simulink model "FaultedPMSM"  (R2023a)
settings: Solver=VariableStepAuto  StartTime=0.0  StopTime=1  MaxStep=1e-4  RelTol=1e-3  AbsTol=1e-3
PreLoadFcn:
  | FaultedPMSMParameters;
undefined symbols (not defined in the file or in its folder): J, RL, Rs, Rsl, Rw, Ry
libraries: fl_lib x45, ee_lib x19, nesl_utility x2
CloseFcn:
  | try close(h1_FaultedPMSM),end
  | clear h1_FaultedPMSM
  | 
  | clear B0    Ld    Npp   Nws   RL    Rsl   Ry
  | clear  g     gT    l     mu0   r     wS
  | clear J   Lq    Ns    PHI   Rs    Rw    csaT
  | clear gS    gY    lm    mur   rY    wY
  | clear gWinding L0 InitialRotorAnglePMSM
  | 
  | clear simlog_FaultedPMSM tout
Description:
  | PMSM with Thermal Model
settings Model: Creator=The MathWorks, Inc.  LastModifiedBy=Derrick Baalaboore
settings SolverCC: AutoScaleAbsTol=off  AlgebraicLoopSolver=TrustRegion
settings DataIOCC: MaxDataPoints=210000  SaveFormat=Array  ReturnWorkspaceOutputs=off  SignalLoggingName=logsout_PMSMWithThermal
settings OptimizationCC: BlockReduction=off  BooleanDataType=off  ReuseModelBlockBuffer=off  LifeSpan=inf
settings DebuggingCC: SaveWithParameterizedLinksMsg=none  UnderspecifiedInitializationDetection=Classic  MergeDetectMultiDrivingBlocksExec=none  SignalResolutionControl=TryResolveAllWithWarning  UnconnectedInputMsg=warning  UnconnectedOutputMsg=warning  UnconnectedLineMsg=warning  AllowSymbolicDim=off  SFUnexpectedBacktrackingDiag=warning  SFNoUnconditionalDefaultTransitionDiag=warning  SFExecutionAtInitializationDiag=none  ArithmeticOperatorsInVariantConditions=warning
settings HardwareCC: ProdBitPerPointer=32  ProdBitPerSizeT=32  ProdBitPerPtrDiffT=32  ProdLargestAtomicFloat=None  ProdIntDivRoundTo=Undefined  ProdEndianess=Unspecified  ProdWordSize=32  ProdHWDeviceType=32-bit Generic  TargetUnknown=on
settings ModelReferenceCC: EnableRefExpFcnMdlSchedulingChecks=on  PropagateSignalLabelsOutOfModel=off
settings SFSimCC: SimUseLocalCustomCode=off  CustomCodeUndefinedFunction=UseInterfaceOnly
settings RTWCC: RTWUseLocalCustomCode=off  DLArmComputeVersion=19.05
settings CodeAppCC: StateflowObjectComments=on
settings GRTTargetCC: TargetLangStandard=C89/C90 (ANSI)
settings ConfigComp: CovMetricSettings=dw  CovSaveCumulativeToWorkspaceVar=on  CovSaveSingleToWorkspaceVar=on  CovExternalEMLEnable=off  CovSFcnEnable=off
settings SimscapeCC: SimscapeLogType=all  SimscapeLogName=simlog_FaultedPMSM  SimscapeLogDecimation=10  SimscapeLogDataHistory=50000

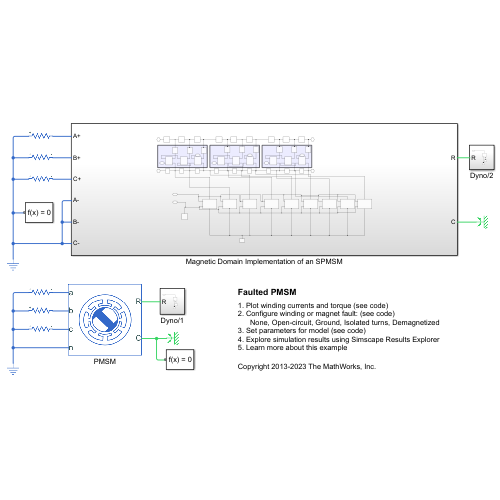
[thumbnail: Simulink's stored preview of the top-level diagram]
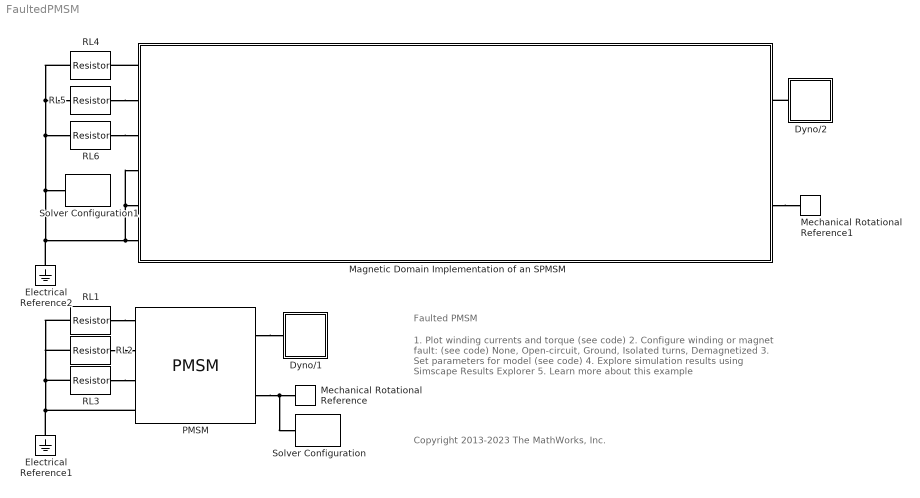
== system FaultedPMSM ==
  note: Faulted PMSM
  note: 1. Plot winding currents and torque (see code)
      | 2. Configure winding or magnet fault: (see code)
      |       None, Open-circuit, Ground, Isolated turns, Demagnetized
      | 3. Set parameters for model (see code)
      | 4. Explore simulation results using Simscape Results Explorer
      | 5. Learn more about this example
  note: Copyright 2013-2023 The MathWorks, Inc.
  Dyno/1 : Subsystem
  Dyno/2 : Subsystem
  Electrical Reference1 : fl_lib/Electrical/Electrical Elements/Electrical Reference
  Electrical Reference2 : fl_lib/Electrical/Electrical Elements/Electrical Reference
  Magnetic Domain Implementation of an SPMSM : Subsystem
  Mechanical Rotational Reference : fl_lib/Mechanical/Rotational Elements/Mechanical Rotational Reference
  Mechanical Rotational Reference1 : fl_lib/Mechanical/Rotational Elements/Mechanical Rotational Reference
  PMSM : ee_lib/Electromechanical/Permanent Magnet/PMSM  port_option=ee.enum.threePhasePort.expanded  winding_type=ee.enum.statorconnection.wye  machine_param=ee.enum.pmsm.parameterization.constant  nPolePairs=Npp  pmflux_param=ee.enum.pmflux.fluxlinkage  pm_flux_linkage=PHI Wb  torque_constant=0.18 N*m/A  back_emf_constant=0.18 V/(rad/s)  stator_param=ee.enum.statorparam.LdLqL0  Ld=Ld H  Lq=Lq H  idVec=[-200, 0, 200] A  iqVec=[-200, 0, 200] A  LdMatrix=0.0002 * ones(3, 3) H  LqMatrix=0.0002 * ones(3, 3) H  PmMatrix=0.1 * ones(3, 3) Wb  ktMatrix=0.18 * ones(3, 3) N*m/A  keMatrix=0.18 * ones(3, 3) V/(rad/s)  L0=L0 H  Ls=0.0002 H  Lm=-0.00002 H  Ms=0.00002 H  Rs=Rw Ohm  zero_sequence=ee.enum.park.zerosequence.include  axes_param=ee.enum.rotorangle.daxis  loss_param=ee.enum.ironloss.none  losses_oc=[0, 0, 0] W  losses_sc=[0, 0, 0] W  f_losses=60 Hz  Isc_losses=95 A  J=J kg*m^2  lam=0 N*m/(rad/s)  i_d_specify=off  i_d_priority=High  i_d=0 A  i_d_nominal_specify=off  i_d_nominal_unit=A  i_d_nominal_value=1  i_q_specify=off  i_q_priority=High  i_q=0 A  i_q_nominal_specify=off  i_q_nominal_unit=A  i_q_nominal_value=1  torque_specify=off  torque_priority=None  torque=0 N*m  torque_nominal_specify=off  torque_nominal_unit=N*m  torque_nominal_value=1  angular_velocity_specify=on  angular_velocity_priority=None  angular_velocity=0 rpm  angular_velocity_nominal_specify=off  angular_velocity_nominal_unit=rpm  angular_velocity_nominal_value=1  angular_position_specify=on  angular_position_priority=High  angular_position=InitialRotorAnglePMSM deg  angular_position_nominal_specify=off  angular_position_nominal_unit=deg  angular_position_nominal_value=1  alpha=3.93e-3 1/K  alpha_flux=-0.001 1/K  Tmeas=298.15 K  stator_thermal_mass=100 J/K  rotor_thermal_mass=200 J/K  Rm_percent_rotor=90  Rd_percent_rotor=30  temperatureA_specify=off  temperatureA_priority=High  temperatureA=25 degC  temperatureA_nominal_specify=off  temperatureA_nominal_unit=degC  temperatureA_nominal_value=1  temperatureB_specify=off  temperatureB_priority=High  temperatureB=25 degC  temperatureB_nominal_specify=off  temperatureB_nominal_unit=degC  temperatureB_nominal_value=1  temperatureC_specify=off  temperatureC_priority=High  temperatureC=25 degC  temperatureC_nominal_specify=off  temperatureC_nominal_unit=degC  temperatureC_nominal_value=1  temperatureR_specify=off  temperatureR_priority=High  temperatureR=25 degC  temperatureR_nominal_specify=off  temperatureR_nominal_unit=degC  temperatureR_nominal_value=1
      settings: InternalSimscapePortConfiguration="{\"Bottom\":[],\"Left\":[{\"id\":\"a\",\"label\":\"a\",\"type\":\"foundation.electrical.electrical\"},{\"id\":\"b\",\"label\":\"b\",\"type\":\"foundation.electrical.electrical\"},{\"id\":\"c\",\"label\":\"c\",\"type\":\"foundation.electrical.electrical\"},{\"id\":\"n\",\"label\":\"n\",\"type\":\"foundation.electrical.electrical\"}],\"Right\":[{\"id\":\"R\",\"label\":\"R\",\"type\":\"foundation.mechanical.rotational.rotational\"},{\"id\":\"C\",\"label\":\"C\",\"type\":\"foundation.mechanical.rotational.rotational\"}],\"Top\":[]}"
  RL1 : fl_lib/Electrical/Electrical Elements/Resistor  R=RL Ohm  i_specify=on  i_priority=High  i=0 A  i_nominal_specify=off  i_nominal_unit=A  i_nominal_value=1  v_specify=off  v_priority=None  v=0 V  v_nominal_specify=off  v_nominal_unit=V  v_nominal_value=1
  RL2 : fl_lib/Electrical/Electrical Elements/Resistor  R=RL Ohm  i_specify=on  i_priority=High  i=0 A  i_nominal_specify=off  i_nominal_unit=A  i_nominal_value=1  v_specify=off  v_priority=None  v=0 V  v_nominal_specify=off  v_nominal_unit=V  v_nominal_value=1
  RL3 : fl_lib/Electrical/Electrical Elements/Resistor  R=RL Ohm  i_specify=on  i_priority=High  i=0 A  i_nominal_specify=off  i_nominal_unit=A  i_nominal_value=1  v_specify=off  v_priority=None  v=0 V  v_nominal_specify=off  v_nominal_unit=V  v_nominal_value=1
  RL4 : fl_lib/Electrical/Electrical Elements/Resistor  R=RL Ohm  i_specify=off  i_priority=High  i=0 A  i_nominal_specify=off  i_nominal_unit=A  i_nominal_value=1  v_specify=off  v_priority=None  v=0 V  v_nominal_specify=off  v_nominal_unit=V  v_nominal_value=1
  RL5 : fl_lib/Electrical/Electrical Elements/Resistor  R=RL Ohm  i_specify=off  i_priority=High  i=0 A  i_nominal_specify=off  i_nominal_unit=A  i_nominal_value=1  v_specify=off  v_priority=None  v=0 V  v_nominal_specify=off  v_nominal_unit=V  v_nominal_value=1
  RL6 : fl_lib/Electrical/Electrical Elements/Resistor  R=RL Ohm  i_specify=off  i_priority=High  i=0 A  i_nominal_specify=off  i_nominal_unit=A  i_nominal_value=1  v_specify=off  v_priority=None  v=0 V  v_nominal_specify=off  v_nominal_unit=V  v_nominal_value=1
  Solver Configuration : nesl_utility/Solver Configuration  PhysicalDomain=network_engine_domain  SubClassName=solver  LeftPortType=input  RightPortType=generic  Tones=[]  Harmonics=[]  SimulateNoise=off  Profile=off  UseLocalSampling=off  EnableSwitchedLinearOptims=on  FrequencyDomain=off  UseCCode=off  RelTol=0.001  AbsTol=1e-06  MinStep=1e-09  ToWorkspace=off  RevertToSquareIcSolve=off  NumHomotopyIterations=100  PhasorMode=off  PhasorModeNumHarmonics=1  ConsistencySolver=NEWTON_FTOL  IndexReductionMethod=DerivativeReplacement  DoDC=off  ResidualTolerance=1e-09  ConsistencyTolSource=GLOBAL  ConsistencyAbsTol=0.001  ConsistencyRelTol=0.001  ConsistencyTolFactor=0.001  UseLocalSolver=off  LocalSolverChoice=NE_BACKWARD_EULER_ADVANCER  ResolveIndetEquations=on  FunctionEvalNumThread=1  LocalSolverSampleTime=0.0001  DoFixedCost=off  MaxNonlinIter=3  MaxModeIter=2  ComputeImpulses=off  ImpulseIterations=1  LinearAlgebra=auto  LinearAlgebraNumThread=0  EquationFormulation=NE_TIME_EF  DelaysMemoryBudget=1024  AutomaticFiltering=on  FilteringTimeConstant=0.001  PartitionStorageMethod=AS_NEEDED  PartitionMemoryBudget=1024  PartitionMethod=ROBUST
  Solver Configuration1 : nesl_utility/Solver Configuration  PhysicalDomain=network_engine_domain  SubClassName=solver  LeftPortType=input  RightPortType=generic  Tones=[]  Harmonics=[]  SimulateNoise=off  Profile=off  UseLocalSampling=off  EnableSwitchedLinearOptims=on  FrequencyDomain=off  UseCCode=off  RelTol=0.001  AbsTol=1e-06  MinStep=1e-09  ToWorkspace=off  RevertToSquareIcSolve=off  NumHomotopyIterations=100  PhasorMode=off  PhasorModeNumHarmonics=1  ConsistencySolver=NEWTON_FTOL  IndexReductionMethod=DerivativeReplacement  DoDC=off  ResidualTolerance=1e-09  ConsistencyTolSource=GLOBAL  ConsistencyAbsTol=0.001  ConsistencyRelTol=0.001  ConsistencyTolFactor=0.001  UseLocalSolver=off  LocalSolverChoice=NE_BACKWARD_EULER_ADVANCER  ResolveIndetEquations=on  FunctionEvalNumThread=1  LocalSolverSampleTime=0.0001  DoFixedCost=off  MaxNonlinIter=3  MaxModeIter=2  ComputeImpulses=off  ImpulseIterations=1  LinearAlgebra=auto  LinearAlgebraNumThread=0  EquationFormulation=NE_TIME_EF  DelaysMemoryBudget=1024  AutomaticFiltering=on  FilteringTimeConstant=0.001  PartitionStorageMethod=AS_NEEDED  PartitionMemoryBudget=1024  PartitionMethod=ROBUST
  connections:
  Electrical Reference1/LConn1 -- PMSM/LConn4 -- RL1/LConn1 -- RL2/LConn1 -- RL3/LConn1
  PMSM/RConn1 -- Dyno/1/LConn1
  RL1/RConn1 -- PMSM/LConn1
  Magnetic Domain Implementation of an SPMSM/RConn2 -- Mechanical Rotational Reference1/LConn1
  RL3/RConn1 -- PMSM/LConn3
  Magnetic Domain Implementation of an SPMSM/LConn1 -- RL4/RConn1
  Dyno/2/LConn1 -- Magnetic Domain Implementation of an SPMSM/RConn1
  PMSM/RConn2 -- Solver Configuration/RConn1 -- Mechanical Rotational Reference/LConn1
  RL2/RConn1 -- PMSM/LConn2
  RL6/RConn1 -- Magnetic Domain Implementation of an SPMSM/LConn3
  RL5/RConn1 -- Magnetic Domain Implementation of an SPMSM/LConn2
  RL4/LConn1 -- Solver Configuration1/RConn1 -- Electrical Reference2/LConn1 -- Magnetic Domain Implementation of an SPMSM/LConn5 -- Magnetic Domain Implementation of an SPMSM/LConn4 -- Magnetic Domain Implementation of an SPMSM/LConn6 -- RL6/LConn1 -- RL5/LConn1

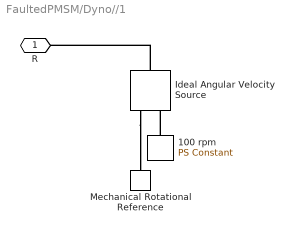
== system FaultedPMSM/Dyno//1 ==
  100 rpm : fl_lib/Physical Signals/Sources/PS Constant  constant=100 rpm
  Ideal Angular Velocity Source : fl_lib/Mechanical/Mechanical Sources/Ideal Angular Velocity Source
  Mechanical Rotational Reference : fl_lib/Mechanical/Rotational Elements/Mechanical Rotational Reference
  R : PMIOPort  Side=Left
  connections:
  Ideal Angular Velocity Source/RConn2 -- Mechanical Rotational Reference/LConn1
  Ideal Angular Velocity Source/LConn1 -- R/RConn1
  100 rpm/RConn1 -- Ideal Angular Velocity Source/RConn1

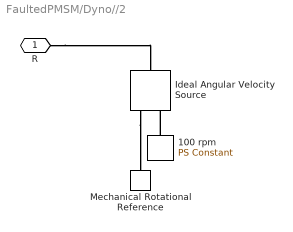
== system FaultedPMSM/Dyno//2 ==
  100 rpm : fl_lib/Physical Signals/Sources/PS Constant  constant=100 rpm
  Ideal Angular Velocity Source : fl_lib/Mechanical/Mechanical Sources/Ideal Angular Velocity Source
  Mechanical Rotational Reference : fl_lib/Mechanical/Rotational Elements/Mechanical Rotational Reference
  R : PMIOPort  Side=Left
  connections:
  100 rpm/RConn1 -- Ideal Angular Velocity Source/RConn1
  Ideal Angular Velocity Source/RConn2 -- Mechanical Rotational Reference/LConn1
  R/RConn1 -- Ideal Angular Velocity Source/LConn1

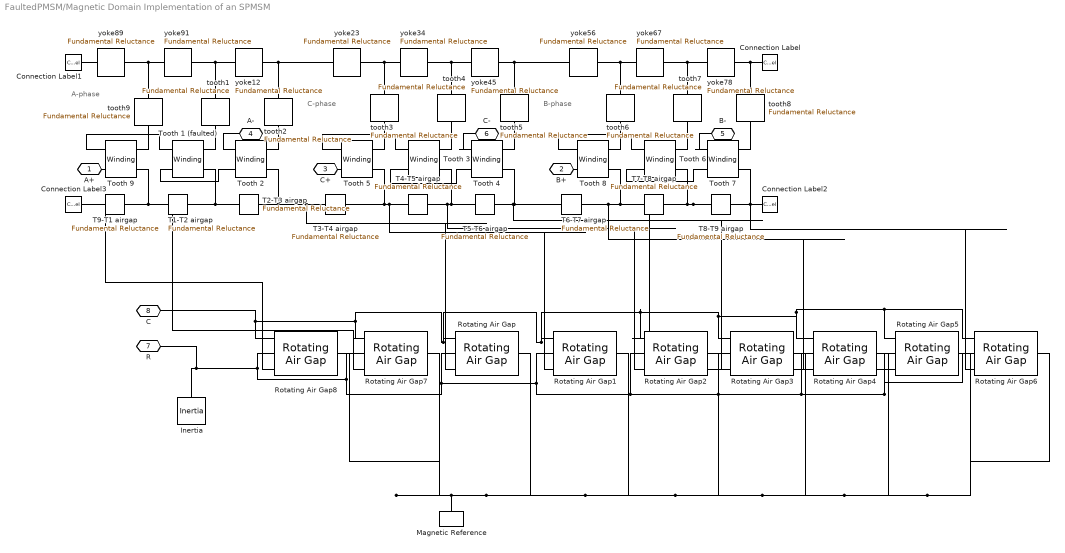
== system FaultedPMSM/Magnetic Domain Implementation of an SPMSM ==
  note: A-phase
  note: C-phase
  note: B-phase
  Connection Label : ConnectionLabel  Label=Y
  Connection Label1 : ConnectionLabel  Label=Y
  Connection Label2 : ConnectionLabel  Label=SL
  Connection Label3 : ConnectionLabel  Label=SL
  Inertia : fl_lib/Mechanical/Rotational Elements/Inertia  inertia=J kg*m^2  num_ports=foundation.enum.numPorts2.one  w_specify=on  w_priority=None  w=0 rad/s  w_nominal_specify=off  w_nominal_unit=rad/s  w_nominal_value=1  t_specify=off  t_priority=High  t=0 N*m  t_nominal_specify=off  t_nominal_unit=N*m  t_nominal_value=1
  Magnetic Reference : fl_lib/Magnetic/Magnetic Elements/Magnetic Reference
      settings: InternalSimscapePortConfiguration="{\"Bottom\":[],\"Left\":[{\"id\":\"M\",\"label\":\"\",\"type\":\"foundation.magnetic.magnetic\"}],\"Right\":[],\"Top\":[]}"
  Rotating Air Gap{,1..8} (9 alike) : ee_lib/Electromechanical/Rotating Air Gap  Nr=5  Ns=9  slot=1  B0=0.4 T  lm=5 mm  mur=1.05  g=1 mm  r=65 mm  l=50 mm  enable_faults=false  lambdaVec=ones(1, 10)  t_fault_transition=100 s  t_fault=1 s  mmf_specify=off  mmf_priority=None  mmf=0 A  mmf_nominal_specify=off  mmf_nominal_unit=A  mmf_nominal_value=1  phi_specify=off  phi_priority=None  phi=0 Wb  phi_nominal_specify=off  phi_nominal_unit=Wb  phi_nominal_value=1  t_specify=off  t_priority=None  t=0 N*m  t_nominal_specify=off  t_nominal_unit=N*m  t_nominal_value=1  w_specify=off  w_priority=None  w=0 rad/s  w_nominal_specify=off  w_nominal_unit=rad/s  w_nominal_value=1  rotorAngle_specify=off  rotorAngle_priority=High  rotorAngle=0 deg  rotorAngle_nominal_specify=off  rotorAngle_nominal_unit=deg  rotorAngle_nominal_value=1
      settings: InternalSimscapePortConfiguration="{\"Bottom\":[{\"id\":\"S\",\"label\":\"S\",\"type\":\"foundation.magnetic.magnetic\"}],\"Left\":[{\"id\":\"C\",\"label\":\"C\",\"type\":\"foundation.mechanical.rotational.rotational\"},{\"id\":\"R\",\"label\":\"R\",\"type\":\"foundation.mechanical.rotational.rotational\"}],\"Right\":[],\"Top\":[{\"id\":\"N\",\"label\":\"N\",\"type\":\"foundation.magnetic.magnetic\"}]}"
  T1-T2 airgap : fl_lib/Magnetic/Magnetic Elements/Fundamental Reluctance  R=Rsl 1/H  phi_specify=off  phi_priority=None  phi=0 Wb  phi_nominal_specify=off  phi_nominal_unit=Wb  phi_nominal_value=1  mmf_specify=off  mmf_priority=None  mmf=0 A  mmf_nominal_specify=off  mmf_nominal_unit=A  mmf_nominal_value=1
      settings: InternalSimscapePortConfiguration="{\"Bottom\":[],\"Left\":[{\"id\":\"N\",\"label\":\"N\",\"type\":\"foundation.magnetic.magnetic\"}],\"Right\":[{\"id\":\"S\",\"label\":\"S\",\"type\":\"foundation.magnetic.magnetic\"}],\"Top\":[]}"
  T2-T3 airgap : fl_lib/Magnetic/Magnetic Elements/Fundamental Reluctance  R=Rsl 1/H  phi_specify=off  phi_priority=None  phi=0 Wb  phi_nominal_specify=off  phi_nominal_unit=Wb  phi_nominal_value=1  mmf_specify=off  mmf_priority=None  mmf=0 A  mmf_nominal_specify=off  mmf_nominal_unit=A  mmf_nominal_value=1
      settings: InternalSimscapePortConfiguration="{\"Bottom\":[],\"Left\":[{\"id\":\"N\",\"label\":\"N\",\"type\":\"foundation.magnetic.magnetic\"}],\"Right\":[{\"id\":\"S\",\"label\":\"S\",\"type\":\"foundation.magnetic.magnetic\"}],\"Top\":[]}"
  T3-T4 airgap : fl_lib/Magnetic/Magnetic Elements/Fundamental Reluctance  R=Rsl 1/H  phi_specify=off  phi_priority=None  phi=0 Wb  phi_nominal_specify=off  phi_nominal_unit=Wb  phi_nominal_value=1  mmf_specify=off  mmf_priority=None  mmf=0 A  mmf_nominal_specify=off  mmf_nominal_unit=A  mmf_nominal_value=1
      settings: InternalSimscapePortConfiguration="{\"Bottom\":[],\"Left\":[{\"id\":\"N\",\"label\":\"N\",\"type\":\"foundation.magnetic.magnetic\"}],\"Right\":[{\"id\":\"S\",\"label\":\"S\",\"type\":\"foundation.magnetic.magnetic\"}],\"Top\":[]}"
  T4-T5 airgap : fl_lib/Magnetic/Magnetic Elements/Fundamental Reluctance  R=Rsl 1/H  phi_specify=off  phi_priority=None  phi=0 Wb  phi_nominal_specify=off  phi_nominal_unit=Wb  phi_nominal_value=1  mmf_specify=off  mmf_priority=None  mmf=0 A  mmf_nominal_specify=off  mmf_nominal_unit=A  mmf_nominal_value=1
      settings: InternalSimscapePortConfiguration="{\"Bottom\":[],\"Left\":[{\"id\":\"N\",\"label\":\"N\",\"type\":\"foundation.magnetic.magnetic\"}],\"Right\":[{\"id\":\"S\",\"label\":\"S\",\"type\":\"foundation.magnetic.magnetic\"}],\"Top\":[]}"
  T5-T6 airgap : fl_lib/Magnetic/Magnetic Elements/Fundamental Reluctance  R=Rsl 1/H  phi_specify=off  phi_priority=None  phi=0 Wb  phi_nominal_specify=off  phi_nominal_unit=Wb  phi_nominal_value=1  mmf_specify=off  mmf_priority=None  mmf=0 A  mmf_nominal_specify=off  mmf_nominal_unit=A  mmf_nominal_value=1
      settings: InternalSimscapePortConfiguration="{\"Bottom\":[],\"Left\":[{\"id\":\"N\",\"label\":\"N\",\"type\":\"foundation.magnetic.magnetic\"}],\"Right\":[{\"id\":\"S\",\"label\":\"S\",\"type\":\"foundation.magnetic.magnetic\"}],\"Top\":[]}"
  T6-T7 airgap : fl_lib/Magnetic/Magnetic Elements/Fundamental Reluctance  R=Rsl 1/H  phi_specify=off  phi_priority=None  phi=0 Wb  phi_nominal_specify=off  phi_nominal_unit=Wb  phi_nominal_value=1  mmf_specify=off  mmf_priority=None  mmf=0 A  mmf_nominal_specify=off  mmf_nominal_unit=A  mmf_nominal_value=1
      settings: InternalSimscapePortConfiguration="{\"Bottom\":[],\"Left\":[{\"id\":\"N\",\"label\":\"N\",\"type\":\"foundation.magnetic.magnetic\"}],\"Right\":[{\"id\":\"S\",\"label\":\"S\",\"type\":\"foundation.magnetic.magnetic\"}],\"Top\":[]}"
  T7-T8 airgap : fl_lib/Magnetic/Magnetic Elements/Fundamental Reluctance  R=Rsl 1/H  phi_specify=off  phi_priority=None  phi=0 Wb  phi_nominal_specify=off  phi_nominal_unit=Wb  phi_nominal_value=1  mmf_specify=off  mmf_priority=None  mmf=0 A  mmf_nominal_specify=off  mmf_nominal_unit=A  mmf_nominal_value=1
      settings: InternalSimscapePortConfiguration="{\"Bottom\":[],\"Left\":[{\"id\":\"N\",\"label\":\"N\",\"type\":\"foundation.magnetic.magnetic\"}],\"Right\":[{\"id\":\"S\",\"label\":\"S\",\"type\":\"foundation.magnetic.magnetic\"}],\"Top\":[]}"
  T8-T9 airgap : fl_lib/Magnetic/Magnetic Elements/Fundamental Reluctance  R=Rsl 1/H  phi_specify=off  phi_priority=None  phi=0 Wb  phi_nominal_specify=off  phi_nominal_unit=Wb  phi_nominal_value=1  mmf_specify=off  mmf_priority=None  mmf=0 A  mmf_nominal_specify=off  mmf_nominal_unit=A  mmf_nominal_value=1
      settings: InternalSimscapePortConfiguration="{\"Bottom\":[],\"Left\":[{\"id\":\"N\",\"label\":\"N\",\"type\":\"foundation.magnetic.magnetic\"}],\"Right\":[{\"id\":\"S\",\"label\":\"S\",\"type\":\"foundation.magnetic.magnetic\"}],\"Top\":[]}"
  T9-T1 airgap : fl_lib/Magnetic/Magnetic Elements/Fundamental Reluctance  R=Rsl 1/H  phi_specify=off  phi_priority=None  phi=0 Wb  phi_nominal_specify=off  phi_nominal_unit=Wb  phi_nominal_value=1  mmf_specify=off  mmf_priority=None  mmf=0 A  mmf_nominal_specify=off  mmf_nominal_unit=A  mmf_nominal_value=1
      settings: InternalSimscapePortConfiguration="{\"Bottom\":[],\"Left\":[{\"id\":\"N\",\"label\":\"N\",\"type\":\"foundation.magnetic.magnetic\"}],\"Right\":[{\"id\":\"S\",\"label\":\"S\",\"type\":\"foundation.magnetic.magnetic\"}],\"Top\":[]}"
  Tooth 1 (faulted) : ee_lib/Passive/Winding  Nw=Nws  Rw=Rw/3 Ohm  Rl=inf 1/H  Gw=gWinding 1/Ohm  thermalPort=simscape.enum.thermaleffects.omit  alpha=3.93e-3 1/K  Tmeas=25 degC  winding_thermal_mass=100 J/K  enable_faults=ee.enum.enable.no  fault_action=simscape.enum.assert.action.none  lambdaPercent=50  turnsShort=ee.enum.faults.faultTurnsShort.no  openCct=ee.enum.faults.faultTurnsOpenCkt.no  groundShort=ee.enum.faults.faultTurnsGroundShort.no  groundShortG=1000 1/Ohm  tau_fault=1e-3 s  fault_trigger=ee.enum.faults.faultTrigger.temporal  t_fault=0.5 s  max_permissible_voltage=100 V  n_fail_on_voltage=1  max_permissible_current=1 A  t_fail_on_current=1 s  T_specify=off  T_priority=None  T=25 degC  T_nominal_specify=off  T_nominal_unit=degC  T_nominal_value=1  i_specify=off  i_priority=None  i=0 A  i_nominal_specify=off  i_nominal_unit=A  i_nominal_value=1  v_specify=off  v_priority=High  v=0 V  v_nominal_specify=off  v_nominal_unit=V  v_nominal_value=1  phi_specify=off  phi_priority=None  phi=0 Wb  phi_nominal_specify=off  phi_nominal_unit=Wb  phi_nominal_value=1  faulted_specify=off  faulted_priority=None  faulted=0  iterm_p_specify=off  iterm_p_priority=None  iterm_p=0 A  iterm_p_nominal_specify=off  iterm_p_nominal_unit=A  iterm_p_nominal_value=1  iterm_n_specify=off  iterm_n_priority=None  iterm_n=0 A  iterm_n_nominal_specify=off  iterm_n_nominal_unit=A  iterm_n_nominal_value=1  power_dissipated_specify=off  power_dissipated_priority=None  power_dissipated=0 W  power_dissipated_nominal_specify=off  power_dissipated_nominal_unit=W  power_dissipated_nominal_value=1
      settings: InternalSimscapePortConfiguration="{\"Bottom\":[],\"Left\":[{\"id\":\"p\",\"label\":\"+\",\"type\":\"foundation.electrical.electrical\"},{\"id\":\"n\",\"label\":\"-\",\"type\":\"foundation.electrical.electrical\"}],\"Right\":[{\"id\":\"N\",\"label\":\"N\",\"type\":\"foundation.magnetic.magnetic\"},{\"id\":\"S\",\"label\":\"S\",\"type\":\"foundation.magnetic.magnetic\"}],\"Top\":[]}"
  Tooth {2..9} (8 alike) : ee_lib/Passive/Winding  Nw=Nws  Rw=Rw/3 Ohm  Rl=inf 1/H  Gw=gWinding 1/Ohm  thermalPort=simscape.enum.thermaleffects.omit  alpha=3.93e-3 1/K  Tmeas=25 degC  winding_thermal_mass=100 J/K  enable_faults=ee.enum.enable.no  fault_action=simscape.enum.assert.action.none  lambdaPercent=50  turnsShort=ee.enum.faults.faultTurnsShort.no  openCct=ee.enum.faults.faultTurnsOpenCkt.no  groundShort=ee.enum.faults.faultTurnsGroundShort.no  groundShortG=0 1/Ohm  tau_fault=1e-3 s  fault_trigger=ee.enum.faults.faultTrigger.temporal  t_fault=1 s  max_permissible_voltage=100 V  n_fail_on_voltage=1  max_permissible_current=1 A  t_fail_on_current=1 s  T_specify=off  T_priority=None  T=25 degC  T_nominal_specify=off  T_nominal_unit=degC  T_nominal_value=1  i_specify=off  i_priority=None  i=0 A  i_nominal_specify=off  i_nominal_unit=A  i_nominal_value=1  v_specify=off  v_priority=None  v=0 V  v_nominal_specify=off  v_nominal_unit=V  v_nominal_value=1  phi_specify=off  phi_priority=None  phi=0 Wb  phi_nominal_specify=off  phi_nominal_unit=Wb  phi_nominal_value=1  faulted_specify=off  faulted_priority=None  faulted=0  iterm_p_specify=off  iterm_p_priority=None  iterm_p=0 A  iterm_p_nominal_specify=off  iterm_p_nominal_unit=A  iterm_p_nominal_value=1  iterm_n_specify=off  iterm_n_priority=None  iterm_n=0 A  iterm_n_nominal_specify=off  iterm_n_nominal_unit=A  iterm_n_nominal_value=1  power_dissipated_specify=off  power_dissipated_priority=None  power_dissipated=0 W  power_dissipated_nominal_specify=off  power_dissipated_nominal_unit=W  power_dissipated_nominal_value=1
      settings: InternalSimscapePortConfiguration="{\"Bottom\":[],\"Left\":[{\"id\":\"p\",\"label\":\"+\",\"type\":\"foundation.electrical.electrical\"},{\"id\":\"n\",\"label\":\"-\",\"type\":\"foundation.electrical.electrical\"}],\"Right\":[{\"id\":\"N\",\"label\":\"N\",\"type\":\"foundation.magnetic.magnetic\"},{\"id\":\"S\",\"label\":\"S\",\"type\":\"foundation.magnetic.magnetic\"}],\"Top\":[]}"
  tooth{1..9} (9 alike) : fl_lib/Magnetic/Magnetic Elements/Fundamental Reluctance  R=Rs 1/H  phi_specify=off  phi_priority=None  phi=0 Wb  phi_nominal_specify=off  phi_nominal_unit=Wb  phi_nominal_value=1  mmf_specify=off  mmf_priority=None  mmf=0 A  mmf_nominal_specify=off  mmf_nominal_unit=A  mmf_nominal_value=1
      settings: InternalSimscapePortConfiguration="{\"Bottom\":[],\"Left\":[{\"id\":\"N\",\"label\":\"N\",\"type\":\"foundation.magnetic.magnetic\"}],\"Right\":[{\"id\":\"S\",\"label\":\"S\",\"type\":\"foundation.magnetic.magnetic\"}],\"Top\":[]}"
  yoke{12,23,34,45,56,67,78,89,91} (9 alike) : fl_lib/Magnetic/Magnetic Elements/Fundamental Reluctance  R=Ry 1/H  phi_specify=off  phi_priority=None  phi=0 Wb  phi_nominal_specify=off  phi_nominal_unit=Wb  phi_nominal_value=1  mmf_specify=off  mmf_priority=None  mmf=0 A  mmf_nominal_specify=off  mmf_nominal_unit=A  mmf_nominal_value=1
      settings: InternalSimscapePortConfiguration="{\"Bottom\":[],\"Left\":[{\"id\":\"N\",\"label\":\"N\",\"type\":\"foundation.magnetic.magnetic\"}],\"Right\":[{\"id\":\"S\",\"label\":\"S\",\"type\":\"foundation.magnetic.magnetic\"}],\"Top\":[]}"
  A+ : PMIOPort  Side=Left
  B+ : PMIOPort  Port=2  Side=Left
  C+ : PMIOPort  Port=3  Side=Left
  A- : PMIOPort  Port=4  Side=Left
  B- : PMIOPort  Port=5  Side=Left
  C- : PMIOPort  Port=6  Side=Left
  R : PMIOPort  Port=7  Side=Right
  C : PMIOPort  Port=8  Side=Right
  connections:
  yoke91/RConn1 -- yoke12/LConn1 -- tooth1/LConn1
  Tooth 1 (faulted)/RConn2 -- Rotating Air Gap7/LConn3 -- T2-T3 airgap/LConn1 -- T1-T2 airgap/RConn1
  Tooth 2/RConn1 -- tooth2/RConn1
  yoke91/LConn1 -- yoke89/RConn1 -- tooth9/LConn1
  yoke89/LConn1 -- Connection Label1/LConn1
  T9-T1 airgap/LConn1 -- Connection Label3/LConn1
  Tooth 9/LConn2 -- A+/RConn1
  Tooth 9/LConn1 -- Tooth 1 (faulted)/LConn1
  Tooth 1 (faulted)/LConn2 -- Tooth 2/LConn2
  Tooth 2/LConn1 -- A-/RConn1
  Tooth 9/RConn2 -- Rotating Air Gap8/LConn3 -- T9-T1 airgap/RConn1 -- T1-T2 airgap/LConn1
  yoke45/LConn1 -- yoke34/RConn1 -- tooth4/LConn1
  yoke34/LConn1 -- yoke23/RConn1 -- tooth3/LConn1
  yoke45/RConn1 -- yoke56/LConn1 -- tooth5/LConn1
  Tooth 5/LConn2 -- C+/RConn1
  Tooth 3/LConn2 -- Tooth 4/LConn2
  Tooth 5/LConn1 -- Tooth 3/LConn1
  Tooth 4/LConn1 -- C-/RConn1
  yoke78/LConn1 -- yoke67/RConn1 -- tooth7/LConn1
  Tooth 6/RConn2 -- T7-T8 airgap/RConn1 -- Rotating Air Gap5/LConn3 -- T8-T9 airgap/LConn1
  yoke67/LConn1 -- yoke56/RConn1 -- tooth6/LConn1
  tooth8/LConn1 -- yoke78/RConn1 -- Connection Label/LConn1
  Tooth 8/LConn2 -- B+/RConn1
  Tooth 8/LConn1 -- Tooth 6/LConn1
  Tooth 6/LConn2 -- Tooth 7/LConn2
  Tooth 7/LConn1 -- B-/RConn1
  Tooth 1 (faulted)/RConn1 -- tooth1/RConn1
  yoke23/LConn1 -- tooth2/LConn1 -- yoke12/RConn1
  Tooth 5/RConn1 -- tooth3/RConn1
  Tooth 3/RConn1 -- tooth4/RConn1
  Tooth 4/RConn1 -- tooth5/RConn1
  Tooth 8/RConn1 -- tooth6/RConn1
  Tooth 6/RConn1 -- tooth7/RConn1
  Tooth 9/RConn1 -- tooth9/RConn1
  Tooth 7/RConn1 -- tooth8/RConn1
  Magnetic Reference/LConn1 -- Rotating Air Gap6/RConn1 -- Rotating Air Gap5/RConn1 -- Rotating Air Gap4/RConn1 -- Rotating Air Gap3/RConn1 -- Rotating Air Gap2/RConn1 -- Rotating Air Gap1/RConn1 -- Rotating Air Gap/RConn1 -- Rotating Air Gap7/RConn1 -- Rotating Air Gap8/RConn1
  Rotating Air Gap1/LConn2 -- R/RConn1 -- Inertia/LConn1 -- Rotating Air Gap8/LConn2 -- Rotating Air Gap7/LConn2 -- Rotating Air Gap/LConn2 -- Rotating Air Gap2/LConn2 -- Rotating Air Gap3/LConn2 -- Rotating Air Gap4/LConn2 -- Rotating Air Gap6/LConn2 -- Rotating Air Gap5/LConn2
  Rotating Air Gap6/LConn1 -- Rotating Air Gap5/LConn1 -- Rotating Air Gap4/LConn1 -- Rotating Air Gap3/LConn1 -- Rotating Air Gap2/LConn1 -- Rotating Air Gap8/LConn1 -- C/RConn1 -- Rotating Air Gap7/LConn1 -- Rotating Air Gap/LConn1 -- Rotating Air Gap1/LConn1
  Tooth 5/RConn2 -- Rotating Air Gap1/LConn3 -- T4-T5 airgap/LConn1 -- T3-T4 airgap/RConn1
  T3-T4 airgap/LConn1 -- Rotating Air Gap/LConn3 -- Tooth 2/RConn2 -- T2-T3 airgap/RConn1
  Tooth 8/RConn2 -- Rotating Air Gap4/LConn3 -- T6-T7 airgap/RConn1 -- T7-T8 airgap/LConn1
  Tooth 3/RConn2 -- Rotating Air Gap2/LConn3 -- T4-T5 airgap/RConn1 -- T5-T6 airgap/LConn1
  T6-T7 airgap/LConn1 -- Rotating Air Gap3/LConn3 -- T5-T6 airgap/RConn1 -- Tooth 4/RConn2
  T8-T9 airgap/RConn1 -- Rotating Air Gap6/LConn3 -- Connection Label2/LConn1 -- Tooth 7/RConn2
